simulink model "ballbeam_sim"  (Simulink 8.1)
settings: Solver=ode45  StartTime=0.0  StopTime=100  RelTol=1e-3
undefined symbols (not defined in the file or in its folder): AP, ballbeam_ctrl, drawBallBeam, P
settings Model: Creator=beard  LastModifiedBy=jhl48
settings OptimizationCC: InitFltsAndDblsToZero=on
settings DebuggingCC: StrictBusMsg=Warning
settings GRTTargetCC: CodeReplacementLibrary=None  CPPClassGenCompliant=on

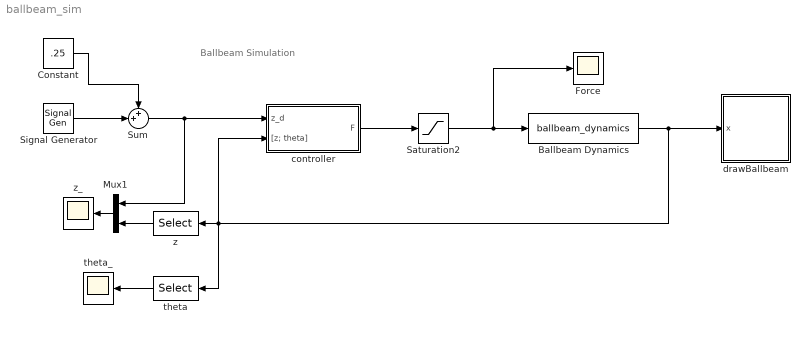
== system ballbeam_sim ==
  note: Ballbeam Simulation
  Ballbeam Dynamics : S-Function  FunctionName=ballbeam_dynamics  Parameters=AP  EnableBusSupport=off
  Constant : Constant  Value=.25
  Force : Scope
      settings: TimeRange=100  YMin=9  YMax=12.25
  Mux1 : Mux  Inputs=2
  Saturation2 : Saturate  UpperLimit=AP.F_max  LowerLimit=-AP.F_max
  Signal Generator : SignalGenerator  WaveForm=square  Amplitude=.125  Frequency=.02
  Sum : Sum  Inputs=++|
  controller : Subsystem
  drawBallbeam : Subsystem
      mask init:
      | % drawing parameters
      | L = 0.5;
      | R = .03;
      mask Display: image(imread('tv.jpg'))
  theta : Selector  InputPortWidth=2  IndexOptions=Index vector (dialog)  Indices=[1]  OutputSizes=1
  theta_ : Scope
      settings: TimeRange=100  YMin=-0.0225  YMax=0.0025
  z : Selector  InputPortWidth=2  IndexOptions=Index vector (dialog)  Indices=[2]  OutputSizes=1
  z_ : Scope
      settings: TimeRange=100  YMin=2.77556e-17  YMax=0.5  SaveName=ScopeData2
  wires:
  Ballbeam Dynamics/1 -> drawBallbeam/1(x), controller/2("[z; theta]"), z/1, theta/1
  controller/1(F) -> Saturation2/1
  Mux1/1 -> z_/1
  Saturation2/1 -> Ballbeam Dynamics/1, Force/1
  z/1 -> Mux1/2
  theta/1 -> theta_/1
  Constant/1 -> Sum/1
  Signal Generator/1 -> Sum/2
  Sum/1 -> Mux1/1, controller/1(z_d)

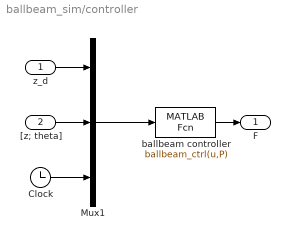
== system ballbeam_sim/controller ==
  z_d : Inport
  "[z; theta]" : Inport  Port=2
  Clock : Clock
  Mux1 : Mux  Inputs=3
  ballbeam controller : MATLABFcn  MATLABFcn=ballbeam_ctrl(u,P)  OutputDimensions=1  SampleTime=P.Ts
  F : Outport
  wires:
  Clock/1 -> Mux1/3
  ballbeam controller/1 -> F/1
  "[z; theta]"/1 -> Mux1/2
  z_d/1 -> Mux1/1
  Mux1/1 -> ballbeam controller/1

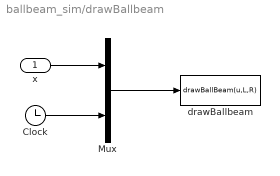
== system ballbeam_sim/drawBallbeam ==
  x : Inport
  Clock : Clock
  Mux : Mux  Inputs=2
  drawBallbeam : MATLABFcn  MATLABFcn=drawBallBeam(u,L,R)  OutputDimensions=0  SampleTime=0.01
  wires:
  Mux/1 -> drawBallbeam/1
  x/1 -> Mux/1
  Clock/1 -> Mux/2
